simulink model "Super12Modif_tmp"  (Simulink 8.3)
settings: Solver=FixedStepDiscrete  StartTime=0.0  StopTime=20.0  RelTol=1e-3
settings Model: Creator=scaife  LastModifiedBy=bourbouh  PauseTimes=10  CovSFcnEnable=on  ExtModeAutoUpdateStatusClock=off
settings DataIOCC: SignalLoggingName=sigsOut
settings DebuggingCC: SaveWithParameterizedLinksMsg=none  SignalResolutionControl=TryResolveAllWithWarning  SolverPrmCheckMsg=none  MultiTaskDSMMsg=warning  MultiTaskCondExecSysMsg=none  FrameProcessingCompatibilityMsg=error  StateNameClashWarn=none
settings HardwareCC: TargetBitPerLong=64  TargetBitPerPointer=64  TargetLongLongMode=on  TargetIntDivRoundTo=Zero  TargetEndianess=LittleEndian  TargetWordSize=64  TargetHWDeviceType=MATLAB Host  ProdEqTarget=off
settings SFSimCC: SimParseCustomCode=off

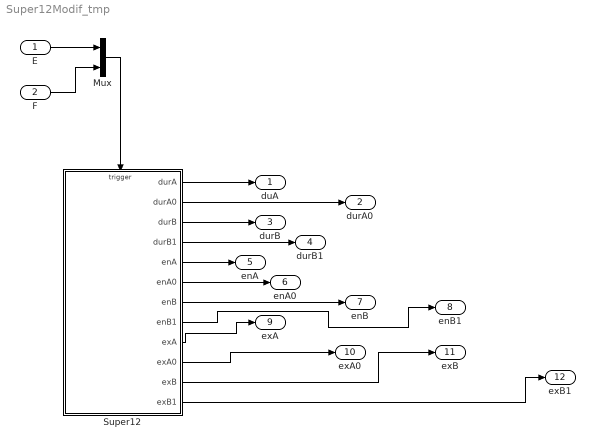
== system Super12Modif_tmp ==
  E : Inport
  F : Inport  Port=2
  Mux : Mux  Inputs=2
  Super12 : Stateflow chart  TreatAsAtomicUnit=on
      settings: PermitHierarchicalResolution=ParametersOnly
  duA : Outport
  durA0 : Outport  Port=2
  durB : Outport  Port=3
  durB1 : Outport  Port=4
  enA : Outport  Port=5
  enA0 : Outport  Port=6
  enB : Outport  Port=7
  enB1 : Outport  Port=8
  exA : Outport  Port=9
  exA0 : Outport  Port=10
  exB : Outport  Port=11
  exB1 : Outport  Port=12
  wires:
  Mux/1 -> Super12/Trigger
  E/1 -> Mux/1
  F/1 -> Mux/2
  Super12/2(durA0) -> durA0/1
  Super12/3(durB) -> durB/1
  Super12/1(durA) -> duA/1
  Super12/4(durB1) -> durB1/1
  Super12/5(enA) -> enA/1
  Super12/6(enA0) -> enA0/1
  Super12/7(enB) -> enB/1
  Super12/8(enB1) -> enB1/1
  Super12/9(exA) -> exA/1
  Super12/12(exB1) -> exB1/1
  Super12/10(exA0) -> exA0/1
  Super12/11(exB) -> exB/1

== stateflow chart Super12 ==
  state A
    entry : enA++
    ex : exA++
    during : durA++
    state A0
      en : enA0++
      du : durA0++
      ex : exA0++
    state A1
    A1 -> A0 : F
    A0 -> A1 [order 2] : F
    (default) -> A0
  state B
    en : enB++
    du : durB++
    ex : exB++
    state B1
      en : enB1++
      du : durB1++
      ex : exB1++
    state B0
    (default) -> B0
    B0 -> B1 : E
    B1 -> B0 [order 2] : E
  (default) -> A
  A -> B : F
  A0 -> B1 [order 1] : E
  B1 -> A0 [order 1] : F
  data: durA output int32 =0; durA0 output int32 =0; durB output int32 =0; durB1 output int32 =0; enA output int32 =0; enA0 output int32 =0; enB output int32 =0; enB1 output int32 =0; exA output int32 =0; exA0 output int32 =0; exB output int32 =0; exB1 output int32 =0
  events: E input EITHER_EDGE_EVENT; F input EITHER_EDGE_EVENT
